simulink model "pid_flc_picomotor"  (R2014a)
settings: Solver=ode45  StartTime=0.0  StopTime=10.0  RelTol=1e-3
libraries: fuzblock x1, simulink x1
settings Model: Creator=KRISH  LastModifiedBy=KRISH
settings DebuggingCC: SolverPrmCheckMsg=none

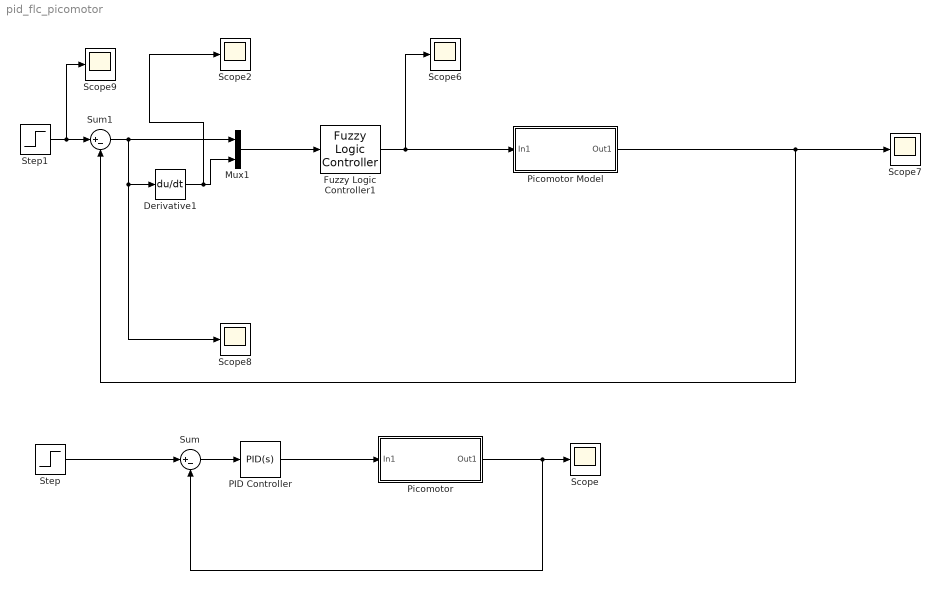
== system pid_flc_picomotor ==
  Derivative1 : Derivative
  Fuzzy Logic Controller1 : fuzblock/Fuzzy Logic  Controller  fis='flc_pid2.fis'
  Mux1 : Mux  Inputs=2
  PID Controller : simulink/Continuous/PID Controller  Controller=PID  TimeDomain=Continuous-time  SampleTime=1  IntegratorMethod=Forward Euler  FilterMethod=Forward Euler  Form=Parallel  P=2.12262361163378  I=105.330786384171  D=0.0105494448840596  N=12185.2047356702  InitialConditionSource=internal  InitialConditionForIntegrator=0  InitialConditionForFilter=0  ExternalReset=none  LimitOutput=off  UpperSaturationLimit=inf  LowerSaturationLimit=-inf  LinearizeAsGain=on  AntiWindupMode=none  Kb=1  TrackingMode=off  Kt=1  PParamMin=[]  PParamMax=[]  IParamMin=[]  IParamMax=[]  DParamMin=[]  DParamMax=[]  NParamMin=[]  NParamMax=[]  KbParamMin=[]  KbParamMax=[]  KtParamMin=[]  KtParamMax=[]  POutMin=[]  POutMax=[]  IOutMin=[]  IOutMax=[]  DOutMin=[]  DOutMax=[]  NOutMin=[]  NOutMax=[]  KbOutMin=[]  KbOutMax=[]  KtOutMin=[]  KtOutMax=[]  IntegratorOutMin=[]  IntegratorOutMax=[]  FilterOutMin=[]  FilterOutMax=[]  SumOutMin=[]  SumOutMax=[]  SumI1OutMin=[]  SumI1OutMax=[]  SumI2OutMin=[]  SumI2OutMax=[]  SumI3OutMin=[]  SumI3OutMax=[]  SumDOutMin=[]  SumDOutMax=[]  SaturationOutMin=[]  SaturationOutMax=[]  IntegratorContinuousStateAttributes=''  IntegratorStateMustResolveToSignalObject=off  IntegratorRTWStateStorageClass=Auto  FilterContinuousStateAttributes=''  FilterStateMustResolveToSignalObject=off  FilterRTWStateStorageClass=Auto
  "Picomotor " : Subsystem
  "Picomotor Model " : Subsystem
  Scope{,2,6..9} (6 alike) : Scope
      Scope settings: YMin=-1.6  YMax=0.3
      Scope2 settings: SaveName=ScopeData2
      Scope6 settings: TimeRange=0.4499999999999993  YMin=0  YMax=0.8  SaveName=ScopeData6
      Scope7 settings: SaveName=ScopeData7
      Scope8 settings: SaveName=ScopeData8
      Scope9 settings: YMin=0.9  YMax=0.9  SaveName=ScopeData9
  Step : Step  Before=-6  After=6  SampleTime=2  VectorParams1D=off  ZeroCross=off
  Step1 : Step  Time=5  Before=-6  After=6  SampleTime=2  VectorParams1D=off  ZeroCross=off
  Sum : Sum  Inputs=|+-
  Sum1 : Sum  Inputs=|+-
  wires:
  Step/1 -> Sum/1
  Sum/1 -> PID Controller/1
  PID Controller/1 -> "Picomotor "/1(In1)
  "Picomotor "/1(Out1) -> Sum/2, Scope/1
  Sum1/1 -> Scope8/1, Derivative1/1, Mux1/1
  Derivative1/1 -> Scope2/1, Mux1/2
  Mux1/1 -> Fuzzy Logic Controller1/1
  Fuzzy Logic Controller1/1 -> "Picomotor Model "/1(In1), Scope6/1
  Step1/1 -> Scope9/1, Sum1/1
  "Picomotor Model "/1(Out1) -> Sum1/2, Scope7/1

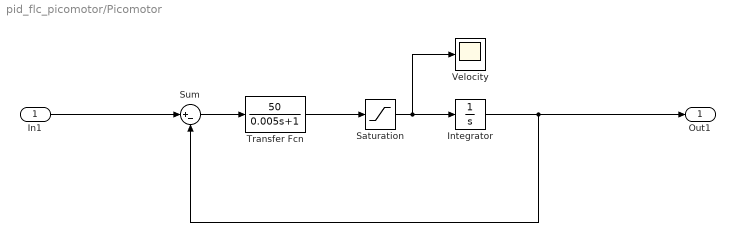
== system pid_flc_picomotor/Picomotor  ==
  In1 : Inport  OutMin=-6  OutMax=6
  Integrator : Integrator
  Saturation : Saturate
  Sum : Sum  Inputs=|+-
  Transfer Fcn : TransferFcn  Numerator=[50]  Denominator=[0.005 1]
  Velocity : Scope
      settings: TimeRange=10
  Out1 : Outport
  wires:
  Transfer Fcn/1 -> Saturation/1
  Saturation/1 -> Velocity/1, Integrator/1
  Integrator/1 -> Sum/2, Out1/1
  Sum/1 -> Transfer Fcn/1
  In1/1 -> Sum/1

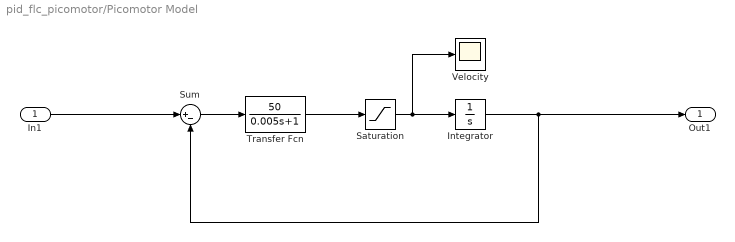
== system pid_flc_picomotor/Picomotor Model  ==
  In1 : Inport  OutMin=-6  OutMax=6
  Integrator : Integrator
  Saturation : Saturate  UpperLimit=6  LowerLimit=-6
  Sum : Sum  Inputs=|+-
  Transfer Fcn : TransferFcn  Numerator=[50]  Denominator=[0.005 1]
  Velocity : Scope
      settings: TimeRange=10
  Out1 : Outport
  wires:
  Transfer Fcn/1 -> Saturation/1
  Saturation/1 -> Velocity/1, Integrator/1
  Integrator/1 -> Sum/2, Out1/1
  Sum/1 -> Transfer Fcn/1
  In1/1 -> Sum/1
